simulink model "ship_p5"  (Simulink 8.5)
settings: Solver=ode45  StartTime=0.0  StopTime=500  RelTol=1e-3
undefined symbols (not defined in the file): A_d, alpha, B_d, C, K_pd, P0_apriori, Q_wd, R_v, T, T_s, task, task2, x0_apriori
libraries: simulink x1
settings Model: Creator=markh  LastModifiedBy=sindrhan
settings DataIOCC: SignalLoggingName=sigsOut
settings OptimizationCC: ExpressionDepthLimit=128  InitFltsAndDblsToZero=on
settings DebuggingCC: SaveWithParameterizedLinksMsg=none  SignalResolutionControl=TryResolveAllWithWarning  MultiTaskDSMMsg=warning  MultiTaskCondExecSysMsg=none  FcnCallInpInsideContextMsg=UseLocalSettings
settings HardwareCC: TargetUnknown=on
settings GRTTargetCC: TargetFcnLib=ansi_tfl_tmw.mat

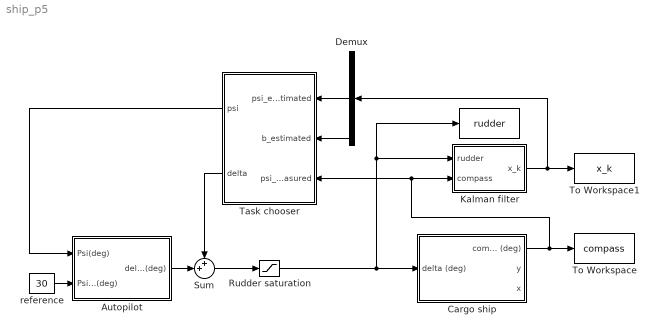
== system ship_p5 ==
  " " : ToWorkspace  VariableName=rudder  SaveFormat=Timeseries  SampleTime=-1
  Autopilot : Subsystem
  Cargo ship : Subsystem  mask(Simple shipmodel for a cargo ship){noise=on, current=on, waves=on}
      mask prompts: noise "measurement noise"
      mask help:
      | Measurement noise:
      | 	checked = noise on
      | 	unchecked = noise off
      |
      | Current:
      | 	checked = current on
      | 	unchecked = current off
      |
      | Waves:
      | 	checked = waves on
      | 	unchecked = waves off
      |
      | Author: Jørgen Spjøtvold, 9/10-2003
      | TTK 4115 Linear system theory.
      | Modified by Jostein Bakkeheim 26/10-2006
  Demux : Demux  Outputs=5
  Kalman filter : Subsystem
  Rudder saturation : Saturate  UpperLimit=45  LowerLimit=-45
  Sum : Sum  Inputs=++|
  Task chooser : Subsystem
  To Workspace : ToWorkspace  VariableName=compass  SaveFormat=Timeseries  SampleTime=-1
  To Workspace1 : ToWorkspace  VariableName=x_k  SaveFormat=Structure With Time  SampleTime=-1
  reference : Constant  Value=30
  wires:
  reference/1 -> Autopilot/2(Psi_r(deg))
  Kalman filter/1(x_k) -> To Workspace1/1, Demux/1
  Rudder saturation/1 -> Cargo ship/1(delta (deg)), " "/1, Kalman filter/1(rudder)
  Cargo ship/1(compass (deg)) -> To Workspace/1, Kalman filter/2(compass), Task chooser/3(psi_measured)
  Sum/1 -> Rudder saturation/1
  Autopilot/1(delta(deg)) -> Sum/2
  Demux/3 -> Task chooser/1(psi_estimated)
  Demux/5 -> Task chooser/2(b_estimated)
  Task chooser/1(psi) -> Autopilot/1(Psi(deg))
  Task chooser/2(delta) -> Sum/1

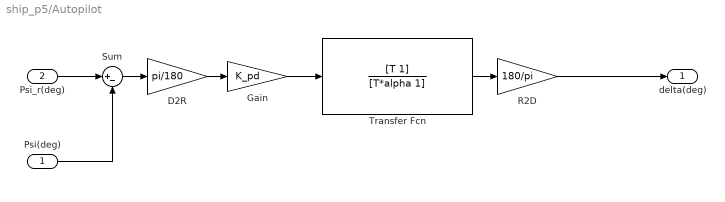
== system ship_p5/Autopilot ==
  Psi(deg) : Inport
  Psi_r(deg) : Inport  Port=2
  D2R : Gain  Gain=pi/180
  Gain : Gain  Gain=K_pd
  R2D : Gain  Gain=180/pi
  Sum : Sum  Inputs=|+-
  Transfer Fcn : TransferFcn  Numerator=[T 1]  Denominator=[T*alpha 1]
  delta(deg) : Outport
  wires:
  Psi_r(deg)/1 -> Sum/1
  Psi(deg)/1 -> Sum/2
  Gain/1 -> Transfer Fcn/1
  Sum/1 -> D2R/1
  D2R/1 -> Gain/1
  Transfer Fcn/1 -> R2D/1
  R2D/1 -> delta(deg)/1

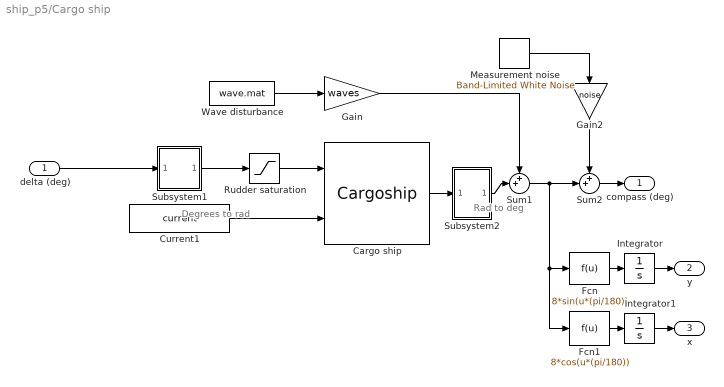
== system ship_p5/Cargo ship ==
  note: Degrees to rad
  note: Rad to deg
  delta (deg) : Inport
  Cargo ship : S-Function  FunctionName=Cargoship  mask(Cargo ship){}
      mask help:
      | S-function which simulates a cargo ship.
      |
      | Author: Jørgen Spjøtvold
      | 20.10-2003
      | Modified by Jostein Bakkeheim 27.10.2006
  Current1 : Constant  Value=current
  Fcn : Fcn  Expr=8*sin(u*(pi/180))
  Fcn1 : Fcn  Expr=8*cos(u*(pi/180))
  Gain : Gain  Gain=waves  SaturateOnIntegerOverflow=on  OutDataTypeStr=Inherit: Same as input  ParamDataTypeStr=Inherit: Same as input
  Gain2 : Gain  Gain=noise  SaturateOnIntegerOverflow=on  OutDataTypeStr=Inherit: Same as input  ParamDataTypeStr=Inherit: Same as input
  Integrator : Integrator
  Integrator1 : Integrator
  Measurement noise : simulink/Sources/Band-Limited White Noise  Cov=[0.001]  Ts=.5  seed=[23341]
  Rudder saturation : Saturate  UpperLimit=45*(pi/180)  LowerLimit=-45*(pi/180)
  Subsystem1 : Subsystem  mask(degrees to radians){}
      mask help: Converts degrees to radians
      mask Display: fprintf('D2R');
  Subsystem2 : Subsystem  mask(radians to degrees){}
      mask help: Converts radians to degrees
      mask Display: fprintf('R2D');
  Sum1 : Sum  Inputs=++|  SaturateOnIntegerOverflow=on
  Sum2 : Sum  Inputs=++|  SaturateOnIntegerOverflow=on
  Wave disturbance : FromFile  FileName=wave.mat  SampleTime=0
  compass (deg) : Outport
  y : Outport  Port=2
  x : Outport  Port=3
  wires:
  delta (deg)/1 -> Subsystem1/1(In1)
  Fcn/1 -> Integrator/1
  Integrator/1 -> y/1
  Fcn1/1 -> Integrator1/1
  Integrator1/1 -> x/1
  Wave disturbance/1 -> Gain/1
  Subsystem2/1(Out1) -> Sum1/2
  Gain/1 -> Sum1/1
  Sum1/1 -> Fcn/1, Fcn1/1, Sum2/2
  Cargo ship/1 -> Subsystem2/1(In1)
  Subsystem1/1(Out1) -> Rudder saturation/1
  Rudder saturation/1 -> Cargo ship/1
  Sum2/1 -> compass (deg)/1
  Measurement noise/1 -> Gain2/1
  Gain2/1 -> Sum2/1
  Current1/1 -> Cargo ship/2

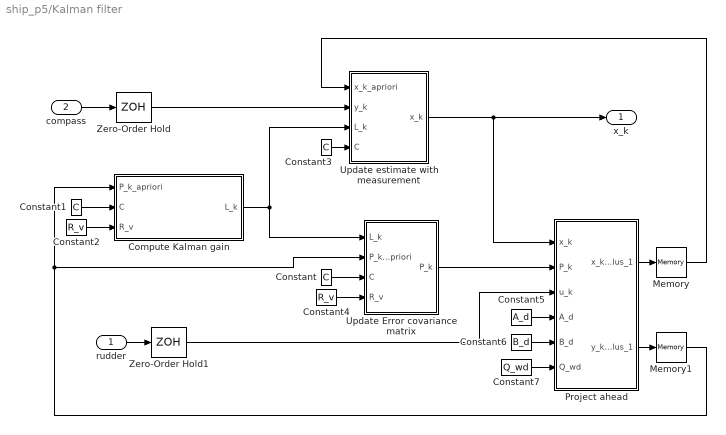
== system ship_p5/Kalman filter ==
  rudder : Inport
  compass : Inport  Port=2
  Compute Kalman gain : MATLAB Function  TreatAsAtomicUnit=on
  Constant : Constant  Value=C  VectorParams1D=off
  Constant1 : Constant  Value=C  VectorParams1D=off
  Constant2 : Constant  Value=R_v
  Constant3 : Constant  Value=C  VectorParams1D=off
  Constant4 : Constant  Value=R_v
  Constant5 : Constant  Value=A_d  VectorParams1D=off
  Constant6 : Constant  Value=B_d  VectorParams1D=off
  Constant7 : Constant  Value=Q_wd  VectorParams1D=off
  Memory : Memory  X0=x0_apriori
  Memory1 : Memory  X0=P0_apriori
  Project ahead : MATLAB Function  TreatAsAtomicUnit=on
  Update Error covariance matrix : MATLAB Function  TreatAsAtomicUnit=on
  Update estimate with measurement : MATLAB Function  TreatAsAtomicUnit=on
  Zero-Order Hold : ZeroOrderHold  SampleTime=T_s
  Zero-Order Hold1 : ZeroOrderHold  SampleTime=T_s
  x_k : Outport
  wires:
  compass/1 -> Zero-Order Hold/1
  rudder/1 -> Zero-Order Hold1/1
  Zero-Order Hold/1 -> Update estimate with measurement/2(y_k)
  Compute Kalman gain/1(L_k) -> Update estimate with measurement/3(L_k), Update Error covariance matrix/1(L_k)
  Zero-Order Hold1/1 -> Project ahead/3(u_k)
  Project ahead/1(x_k_plus_1) -> Memory/1
  Project ahead/2(y_k_plus_1) -> Memory1/1
  Memory/1 -> Update estimate with measurement/1(x_k_apriori)
  Memory1/1 -> Update Error covariance matrix/2(P_k_apriori), Compute Kalman gain/1(P_k_apriori)
  Update estimate with measurement/1(x_k) -> Project ahead/1(x_k), x_k/1
  Update Error covariance matrix/1(P_k) -> Project ahead/2(P_k)
  Constant/1 -> Update Error covariance matrix/3(C)
  Constant1/1 -> Compute Kalman gain/2(C)
  Constant2/1 -> Compute Kalman gain/3(R_v)
  Constant3/1 -> Update estimate with measurement/4(C)
  Constant4/1 -> Update Error covariance matrix/4(R_v)
  Constant5/1 -> Project ahead/4(A_d)
  Constant6/1 -> Project ahead/5(B_d)
  Constant7/1 -> Project ahead/6(Q_wd)

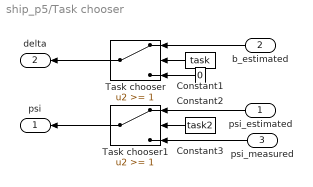
== system ship_p5/Task chooser ==
  psi_estimated : Inport
  b_estimated : Inport  Port=2
  psi_measured : Inport  Port=3
  Constant1 : Constant  Value=task
  Constant2 : Constant  Value=0
  Constant3 : Constant  Value=task2
  Task chooser : Switch  Threshold=1
  Task chooser1 : Switch  Threshold=1
  psi : Outport
  delta : Outport  Port=2
  wires:
  psi_estimated/1 -> Task chooser1/1
  Task chooser/1 -> delta/1
  psi_measured/1 -> Task chooser1/3
  Task chooser1/1 -> psi/1
  Constant3/1 -> Task chooser1/2
  Constant1/1 -> Task chooser/2
  Constant2/1 -> Task chooser/3
  b_estimated/1 -> Task chooser/1

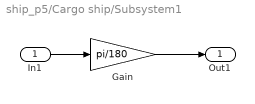
== system ship_p5/Cargo ship/Subsystem1 ==
  In1 : Inport
  Gain : Gain  Gain=pi/180  SaturateOnIntegerOverflow=on  OutDataTypeStr=Inherit: Same as input  ParamDataTypeStr=Inherit: Same as input
  Out1 : Outport
  wires:
  Gain/1 -> Out1/1
  In1/1 -> Gain/1

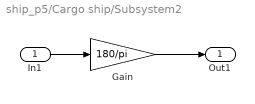
== system ship_p5/Cargo ship/Subsystem2 ==
  In1 : Inport
  Gain : Gain  Gain=180/pi  SaturateOnIntegerOverflow=on  OutDataTypeStr=Inherit: Same as input  ParamDataTypeStr=Inherit: Same as input
  Out1 : Outport
  wires:
  Gain/1 -> Out1/1
  In1/1 -> Gain/1

== matlab function Kalman filter/Update Error covariance matrix ==
  data: L_k input double; P_k output double; P_k_apriori input double; C input double; R_v input double
function P_k = fcn(L_k, P_k_apriori, C, R_v)
P_k = (eye(5) - L_k * C) * P_k_apriori * (eye(5) - L_k * C).' + L_k * R_v * L_k.';

== matlab function Kalman filter/Compute Kalman gain ==
  data: P_k_apriori input double; L_k output double; C input double; R_v input double
function L_k = fcn(P_k_apriori, C, R_v)
L_k = P_k_apriori * C.' * inv(C * P_k_apriori * C.' + R_v);

== matlab function Kalman filter/Update estimate with measurement ==
  data: x_k_apriori input double; x_k output double; y_k input double; L_k input double; C input double
function x_k = fcn(x_k_apriori, y_k, L_k, C)
x_k = x_k_apriori + L_k * (y_k - C * x_k_apriori);

== matlab function Kalman filter/Project ahead ==
  data: x_k input double; x_k_plus_1 output double; y_k_plus_1 output double; P_k input double; u_k input double; A_d input double; B_d input double; Q_wd input double
function [x_k_plus_1,y_k_plus_1] = fcn(x_k, P_k, u_k, A_d, B_d, Q_wd)
x_k_plus_1 = A_d * x_k + B_d * u_k;
y_k_plus_1 = A_d * P_k * A_d.' + Q_wd;
